simulink model "MdXX_RspToNetWork"  (R2024b)
settings: Solver=FixedStepDiscrete  StartTime=0.0  StopTime=10.0  FixedStep=0.01  RelTol=1e-3
(part 2 of 3)

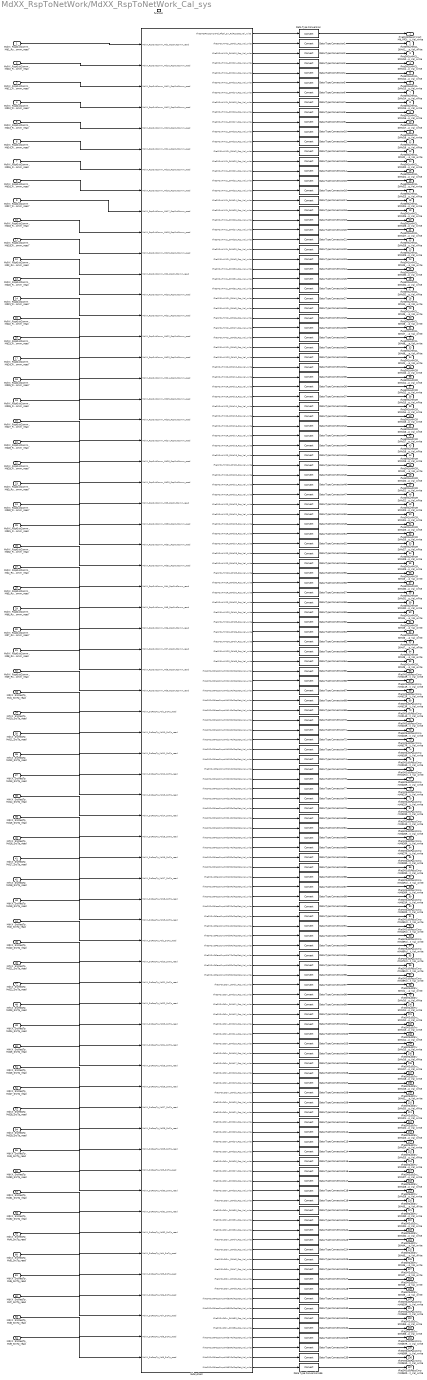
== system MdXX_RspToNetWork/MdXX_RspToNetWork_Cal_sys ==
  MdXX_RspOutComm_Md1_RspOutComm_read : Inport
  MdXX_RspOutComm_Md10_RspOutComm_read : Inport  Port=2
  MdXX_RspOutComm_Md11_RspOutComm_read : Inport  Port=3
  MdXX_RspOutComm_Md12_RspOutComm_read : Inport  Port=4
  MdXX_RspOutComm_Md13_RspOutComm_read : Inport  Port=5
  MdXX_RspOutComm_Md14_RspOutComm_read : Inport  Port=6
  MdXX_RspOutComm_Md15_RspOutComm_read : Inport  Port=7
  MdXX_RspOutComm_Md16_RspOutComm_read : Inport  Port=8
  MdXX_RspOutComm_Md17_RspOutComm_read : Inport  Port=9
  MdXX_RspOutComm_Md18_RspOutComm_read : Inport  Port=10
  MdXX_RspOutComm_Md19_RspOutComm_read : Inport  Port=11
  MdXX_RspOutComm_Md2_RspOutComm_read : Inport  Port=12
  MdXX_RspOutComm_Md20_RspOutComm_read : Inport  Port=13
  MdXX_RspOutComm_Md21_RspOutComm_read : Inport  Port=14
  MdXX_RspOutComm_Md22_RspOutComm_read : Inport  Port=15
  MdXX_RspOutComm_Md23_RspOutComm_read : Inport  Port=16
  MdXX_RspOutComm_Md24_RspOutComm_read : Inport  Port=17
  MdXX_RspOutComm_Md25_RspOutComm_read : Inport  Port=18
  MdXX_RspOutComm_Md26_RspOutComm_read : Inport  Port=19
  MdXX_RspOutComm_Md27_RspOutComm_read : Inport  Port=20
  MdXX_RspOutComm_Md28_RspOutComm_read : Inport  Port=21
  MdXX_RspOutComm_Md29_RspOutComm_read : Inport  Port=22
  MdXX_RspOutComm_Md3_RspOutComm_read : Inport  Port=23
  MdXX_RspOutComm_Md30_RspOutComm_read : Inport  Port=24
  MdXX_RspOutComm_Md31_RspOutComm_read : Inport  Port=25
  MdXX_RspOutComm_Md32_RspOutComm_read : Inport  Port=26
  MdXX_RspOutComm_Md4_RspOutComm_read : Inport  Port=27
  MdXX_RspOutComm_Md5_RspOutComm_read : Inport  Port=28
  MdXX_RspOutComm_Md6_RspOutComm_read : Inport  Port=29
  MdXX_RspOutComm_Md7_RspOutComm_read : Inport  Port=30
  MdXX_RspOutComm_Md8_RspOutComm_read : Inport  Port=31
  MdXX_RspOutComm_Md9_RspOutComm_read : Inport  Port=32
  MdXX_SrcReqTp_Md1_SrcTp_read : Inport  Port=33
  MdXX_SrcReqTp_Md10_SrcTp_read : Inport  Port=34
  MdXX_SrcReqTp_Md11_SrcTp_read : Inport  Port=35
  MdXX_SrcReqTp_Md12_SrcTp_read : Inport  Port=36
  MdXX_SrcReqTp_Md13_SrcTp_read : Inport  Port=37
  MdXX_SrcReqTp_Md14_SrcTp_read : Inport  Port=38
  MdXX_SrcReqTp_Md15_SrcTp_read : Inport  Port=39
  MdXX_SrcReqTp_Md16_SrcTp_read : Inport  Port=40
  MdXX_SrcReqTp_Md17_SrcTp_read : Inport  Port=41
  MdXX_SrcReqTp_Md18_SrcTp_read : Inport  Port=42
  MdXX_SrcReqTp_Md19_SrcTp_read : Inport  Port=43
  MdXX_SrcReqTp_Md2_SrcTp_read : Inport  Port=44
  MdXX_SrcReqTp_Md20_SrcTp_read : Inport  Port=45
  MdXX_SrcReqTp_Md21_SrcTp_read : Inport  Port=46
  MdXX_SrcReqTp_Md22_SrcTp_read : Inport  Port=47
  MdXX_SrcReqTp_Md23_SrcTp_read : Inport  Port=48
  MdXX_SrcReqTp_Md24_SrcTp_read : Inport  Port=49
  MdXX_SrcReqTp_Md25_SrcTp_read : Inport  Port=50
  MdXX_SrcReqTp_Md26_SrcTp_read : Inport  Port=51
  MdXX_SrcReqTp_Md27_SrcTp_read : Inport  Port=52
  MdXX_SrcReqTp_Md28_SrcTp_read : Inport  Port=53
  MdXX_SrcReqTp_Md29_SrcTp_read : Inport  Port=54
  MdXX_SrcReqTp_Md3_SrcTp_read : Inport  Port=55
  MdXX_SrcReqTp_Md30_SrcTp_read : Inport  Port=56
  MdXX_SrcReqTp_Md31_SrcTp_read : Inport  Port=57
  MdXX_SrcReqTp_Md32_SrcTp_read : Inport  Port=58
  MdXX_SrcReqTp_Md4_SrcTp_read : Inport  Port=59
  MdXX_SrcReqTp_Md5_SrcTp_read : Inport  Port=60
  MdXX_SrcReqTp_Md6_SrcTp_read : Inport  Port=61
  MdXX_SrcReqTp_Md7_SrcTp_read : Inport  Port=62
  MdXX_SrcReqTp_Md8_SrcTp_read : Inport  Port=63
  MdXX_SrcReqTp_Md9_SrcTp_read : Inport  Port=64
  function : TriggerPort  TriggerType=function-call  IsSimulinkFunction=on  FunctionName=MdXX_RspToNetWork_Cal  VariantControl=(inherit)
  Data Type Conversion{,1..136} (137 alike) : DataTypeConversion  SaturateOnIntegerOverflow=off  RndMeth=Floor
  Subsystem : Subsystem
  IfVeSMStPassCmprtMd_RfCtrl_Sw_RclRspStat_Val_write : Outport  VectorParamsAs1DForOutWhenUnconnected=off
  IfVeSMSuHMI2L_StMd1_Rsp_Val_write : Outport  Port=2  VectorParamsAs1DForOutWhenUnconnected=off
  IfVeSMSuHMI2L_StMd10_Rsp_Val_write : Outport  Port=3  VectorParamsAs1DForOutWhenUnconnected=off
  IfVeSMSuHMI2L_StMd11_Rsp_Val_write : Outport  Port=4  VectorParamsAs1DForOutWhenUnconnected=off
  IfVeSMSuHMI2L_StMd12_Rsp_Val_write : Outport  Port=5  VectorParamsAs1DForOutWhenUnconnected=off
  IfVeSMSuHMI2L_StMd13_Rsp_Val_write : Outport  Port=6  VectorParamsAs1DForOutWhenUnconnected=off
  IfVeSMSuHMI2L_StMd14_Rsp_Val_write : Outport  Port=7  VectorParamsAs1DForOutWhenUnconnected=off
  IfVeSMSuHMI2L_StMd15_Rsp_Val_write : Outport  Port=8  VectorParamsAs1DForOutWhenUnconnected=off
  IfVeSMSuHMI2L_StMd16_Rsp_Val_write : Outport  Port=9  VectorParamsAs1DForOutWhenUnconnected=off
  IfVeSMSuHMI2L_StMd17_Rsp_Val_write : Outport  Port=10  VectorParamsAs1DForOutWhenUnconnected=off
  IfVeSMSuHMI2L_StMd18_Rsp_Val_write : Outport  Port=11  VectorParamsAs1DForOutWhenUnconnected=off
  IfVeSMSuHMI2L_StMd19_Rsp_Val_write : Outport  Port=12  VectorParamsAs1DForOutWhenUnconnected=off
  IfVeSMSuHMI2L_StMd2_Rsp_Val_write : Outport  Port=13  VectorParamsAs1DForOutWhenUnconnected=off
  IfVeSMSuHMI2L_StMd20_Rsp_Val_write : Outport  Port=14  VectorParamsAs1DForOutWhenUnconnected=off
  IfVeSMSuHMI2L_StMd21_Rsp_Val_write : Outport  Port=15  VectorParamsAs1DForOutWhenUnconnected=off
  IfVeSMSuHMI2L_StMd22_Rsp_Val_write : Outport  Port=16  VectorParamsAs1DForOutWhenUnconnected=off
  IfVeSMSuHMI2L_StMd23_Rsp_Val_write : Outport  Port=17  VectorParamsAs1DForOutWhenUnconnected=off
  IfVeSMSuHMI2L_StMd24_Rsp_Val_write : Outport  Port=18  VectorParamsAs1DForOutWhenUnconnected=off
  IfVeSMSuHMI2L_StMd25_Rsp_Val_write : Outport  Port=19  VectorParamsAs1DForOutWhenUnconnected=off
  IfVeSMSuHMI2L_StMd26_Rsp_Val_write : Outport  Port=20  VectorParamsAs1DForOutWhenUnconnected=off
  IfVeSMSuHMI2L_StMd27_Rsp_Val_write : Outport  Port=21  VectorParamsAs1DForOutWhenUnconnected=off
  IfVeSMSuHMI2L_StMd28_Rsp_Val_write : Outport  Port=22  VectorParamsAs1DForOutWhenUnconnected=off
  IfVeSMSuHMI2L_StMd29_Rsp_Val_write : Outport  Port=23  VectorParamsAs1DForOutWhenUnconnected=off
  IfVeSMSuHMI2L_StMd3_Rsp_Val_write : Outport  Port=24  VectorParamsAs1DForOutWhenUnconnected=off
  IfVeSMSuHMI2L_StMd30_Rsp_Val_write : Outport  Port=25  VectorParamsAs1DForOutWhenUnconnected=off
  IfVeSMSuHMI2L_StMd31_Rsp_Val_write : Outport  Port=26  VectorParamsAs1DForOutWhenUnconnected=off
  IfVeSMSuHMI2L_StMd32_Rsp_Val_write : Outport  Port=27  VectorParamsAs1DForOutWhenUnconnected=off
  IfVeSMSuHMI2L_StMd4_Rsp_Val_write : Outport  Port=28  VectorParamsAs1DForOutWhenUnconnected=off
  IfVeSMSuHMI2L_StMd5_Rsp_Val_write : Outport  Port=29  VectorParamsAs1DForOutWhenUnconnected=off
  IfVeSMSuHMI2L_StMd6_Rsp_Val_write : Outport  Port=30  VectorParamsAs1DForOutWhenUnconnected=off
  IfVeSMSuHMI2L_StMd7_Rsp_Val_write : Outport  Port=31  VectorParamsAs1DForOutWhenUnconnected=off
  IfVeSMSuHMI2L_StMd8_Rsp_Val_write : Outport  Port=32  VectorParamsAs1DForOutWhenUnconnected=off
  IfVeSMSuHMI2L_StMd9_Rsp_Val_write : Outport  Port=33  VectorParamsAs1DForOutWhenUnconnected=off
  IfVeSMSuHMI2R_StMd1_Rsp_Val_write : Outport  Port=34  VectorParamsAs1DForOutWhenUnconnected=off
  IfVeSMSuHMI2R_StMd10_Rsp_Val_write : Outport  Port=35  VectorParamsAs1DForOutWhenUnconnected=off
  IfVeSMSuHMI2R_StMd11_Rsp_Val_write : Outport  Port=36  VectorParamsAs1DForOutWhenUnconnected=off
  IfVeSMSuHMI2R_StMd12_Rsp_Val_write : Outport  Port=37  VectorParamsAs1DForOutWhenUnconnected=off
  IfVeSMSuHMI2R_StMd13_Rsp_Val_write : Outport  Port=38  VectorParamsAs1DForOutWhenUnconnected=off
  IfVeSMSuHMI2R_StMd14_Rsp_Val_write : Outport  Port=39  VectorParamsAs1DForOutWhenUnconnected=off
  IfVeSMSuHMI2R_StMd15_Rsp_Val_write : Outport  Port=40  VectorParamsAs1DForOutWhenUnconnected=off
  IfVeSMSuHMI2R_StMd16_Rsp_Val_write : Outport  Port=41  VectorParamsAs1DForOutWhenUnconnected=off
  IfVeSMSuHMI2R_StMd17_Rsp_Val_write : Outport  Port=42  VectorParamsAs1DForOutWhenUnconnected=off
  IfVeSMSuHMI2R_StMd18_Rsp_Val_write : Outport  Port=43  VectorParamsAs1DForOutWhenUnconnected=off
  IfVeSMSuHMI2R_StMd19_Rsp_Val_write : Outport  Port=44  VectorParamsAs1DForOutWhenUnconnected=off
  IfVeSMSuHMI2R_StMd2_Rsp_Val_write : Outport  Port=45  VectorParamsAs1DForOutWhenUnconnected=off
  IfVeSMSuHMI2R_StMd20_Rsp_Val_write : Outport  Port=46  VectorParamsAs1DForOutWhenUnconnected=off
  IfVeSMSuHMI2R_StMd21_Rsp_Val_write : Outport  Port=47  VectorParamsAs1DForOutWhenUnconnected=off
  IfVeSMSuHMI2R_StMd22_Rsp_Val_write : Outport  Port=48  VectorParamsAs1DForOutWhenUnconnected=off
  IfVeSMSuHMI2R_StMd23_Rsp_Val_write : Outport  Port=49  VectorParamsAs1DForOutWhenUnconnected=off
  IfVeSMSuHMI2R_StMd24_Rsp_Val_write : Outport  Port=50  VectorParamsAs1DForOutWhenUnconnected=off
  IfVeSMSuHMI2R_StMd25_Rsp_Val_write : Outport  Port=51  VectorParamsAs1DForOutWhenUnconnected=off
  IfVeSMSuHMI2R_StMd26_Rsp_Val_write : Outport  Port=52  VectorParamsAs1DForOutWhenUnconnected=off
  IfVeSMSuHMI2R_StMd27_Rsp_Val_write : Outport  Port=53  VectorParamsAs1DForOutWhenUnconnected=off
  IfVeSMSuHMI2R_StMd28_Rsp_Val_write : Outport  Port=54  VectorParamsAs1DForOutWhenUnconnected=off
  IfVeSMSuHMI2R_StMd29_Rsp_Val_write : Outport  Port=55  VectorParamsAs1DForOutWhenUnconnected=off
  IfVeSMSuHMI2R_StMd3_Rsp_Val_write : Outport  Port=56  VectorParamsAs1DForOutWhenUnconnected=off
  IfVeSMSuHMI2R_StMd30_Rsp_Val_write : Outport  Port=57  VectorParamsAs1DForOutWhenUnconnected=off
  IfVeSMSuHMI2R_StMd31_Rsp_Val_write : Outport  Port=58  VectorParamsAs1DForOutWhenUnconnected=off
  IfVeSMSuHMI2R_StMd32_Rsp_Val_write : Outport  Port=59  VectorParamsAs1DForOutWhenUnconnected=off
  IfVeSMSuHMI2R_StMd4_Rsp_Val_write : Outport  Port=60  VectorParamsAs1DForOutWhenUnconnected=off
  IfVeSMSuHMI2R_StMd5_Rsp_Val_write : Outport  Port=61  VectorParamsAs1DForOutWhenUnconnected=off
  IfVeSMSuHMI2R_StMd6_Rsp_Val_write : Outport  Port=62  VectorParamsAs1DForOutWhenUnconnected=off
  IfVeSMSuHMI2R_StMd7_Rsp_Val_write : Outport  Port=63  VectorParamsAs1DForOutWhenUnconnected=off
  IfVeSMSuHMI2R_StMd8_Rsp_Val_write : Outport  Port=64  VectorParamsAs1DForOutWhenUnconnected=off
  IfVeSMSuHMI2R_StMd9_Rsp_Val_write : Outport  Port=65  VectorParamsAs1DForOutWhenUnconnected=off
  IfVeSMSuStPassCmprtMd10RclRspStat_Val_write : Outport  Port=66  VectorParamsAs1DForOutWhenUnconnected=off
  IfVeSMSuStPassCmprtMd11RclRspStat_Val_write : Outport  Port=67  VectorParamsAs1DForOutWhenUnconnected=off
  IfVeSMSuStPassCmprtMd12RclRspStat_Val_write : Outport  Port=68  VectorParamsAs1DForOutWhenUnconnected=off
  IfVeSMSuStPassCmprtMd13RclRspStat_Val_write : Outport  Port=69  VectorParamsAs1DForOutWhenUnconnected=off
  IfVeSMSuStPassCmprtMd14RclRspStat_Val_write : Outport  Port=70  VectorParamsAs1DForOutWhenUnconnected=off
  IfVeSMSuStPassCmprtMd15RclRspStat_Val_write : Outport  Port=71  VectorParamsAs1DForOutWhenUnconnected=off
  IfVeSMSuStPassCmprtMd16RclRspStat_Val_write : Outport  Port=72  VectorParamsAs1DForOutWhenUnconnected=off
  IfVeSMSuStPassCmprtMd17RclRspStat_Val_write : Outport  Port=73  VectorParamsAs1DForOutWhenUnconnected=off
  IfVeSMSuStPassCmprtMd18RclRspStat_Val_write : Outport  Port=74  VectorParamsAs1DForOutWhenUnconnected=off
  IfVeSMSuStPassCmprtMd19RclRspStat_Val_write : Outport  Port=75  VectorParamsAs1DForOutWhenUnconnected=off
  IfVeSMSuStPassCmprtMd1RclRspStat_Val_write : Outport  Port=76  VectorParamsAs1DForOutWhenUnconnected=off
  IfVeSMSuStPassCmprtMd20RclRspStat_Val_write : Outport  Port=77  VectorParamsAs1DForOutWhenUnconnected=off
  IfVeSMSuStPassCmprtMd21RclRspStat_Val_write : Outport  Port=78  VectorParamsAs1DForOutWhenUnconnected=off
  IfVeSMSuStPassCmprtMd22RclRspStat_Val_write : Outport  Port=79  VectorParamsAs1DForOutWhenUnconnected=off
  IfVeSMSuStPassCmprtMd23RclRspStat_Val_write : Outport  Port=80  VectorParamsAs1DForOutWhenUnconnected=off
  IfVeSMSuStPassCmprtMd24RclRspStat_Val_write : Outport  Port=81  VectorParamsAs1DForOutWhenUnconnected=off
  IfVeSMSuStPassCmprtMd25RclRspStat_Val_write : Outport  Port=82  VectorParamsAs1DForOutWhenUnconnected=off
  IfVeSMSuStPassCmprtMd26RclRspStat_Val_write : Outport  Port=83  VectorParamsAs1DForOutWhenUnconnected=off
  IfVeSMSuStPassCmprtMd27RclRspStat_Val_write : Outport  Port=84  VectorParamsAs1DForOutWhenUnconnected=off
  IfVeSMSuStPassCmprtMd28RclRspStat_Val_write : Outport  Port=85  VectorParamsAs1DForOutWhenUnconnected=off
  IfVeSMSuStPassCmprtMd29RclRspStat_Val_write : Outport  Port=86  VectorParamsAs1DForOutWhenUnconnected=off
  IfVeSMSuStPassCmprtMd2RclRspStat_Val_write : Outport  Port=87  VectorParamsAs1DForOutWhenUnconnected=off
  IfVeSMSuStPassCmprtMd30RclRspStat_Val_write : Outport  Port=88  VectorParamsAs1DForOutWhenUnconnected=off
  IfVeSMSuStPassCmprtMd31RclRspStat_Val_write : Outport  Port=89  VectorParamsAs1DForOutWhenUnconnected=off
  IfVeSMSuStPassCmprtMd32RclRspStat_Val_write : Outport  Port=90  VectorParamsAs1DForOutWhenUnconnected=off
  IfVeSMSuStPassCmprtMd3RclRspStat_Val_write : Outport  Port=91  VectorParamsAs1DForOutWhenUnconnected=off
  IfVeSMSuStPassCmprtMd4RclRspStat_Val_write : Outport  Port=92  VectorParamsAs1DForOutWhenUnconnected=off
  IfVeSMSuStPassCmprtMd5RclRspStat_Val_write : Outport  Port=93  VectorParamsAs1DForOutWhenUnconnected=off
  IfVeSMSuStPassCmprtMd6RclRspStat_Val_write : Outport  Port=94  VectorParamsAs1DForOutWhenUnconnected=off
  IfVeSMSuStPassCmprtMd7RclRspStat_Val_write : Outport  Port=95  VectorParamsAs1DForOutWhenUnconnected=off
  IfVeSMSuStPassCmprtMd8RclRspStat_Val_write : Outport  Port=96  VectorParamsAs1DForOutWhenUnconnected=off
  IfVeSMSuStPassCmprtMd9RclRspStat_Val_write : Outport  Port=97  VectorParamsAs1DForOutWhenUnconnected=off
  IfVeSMSuStSrv_StMd1_Rsp_Val_write : Outport  Port=98  VectorParamsAs1DForOutWhenUnconnected=off
  IfVeSMSuStSrv_StMd10_Rsp_Val_write : Outport  Port=99  VectorParamsAs1DForOutWhenUnconnected=off
  IfVeSMSuStSrv_StMd11_Rsp_Val_write : Outport  Port=100  VectorParamsAs1DForOutWhenUnconnected=off
  IfVeSMSuStSrv_StMd12_Rsp_Val_write : Outport  Port=101  VectorParamsAs1DForOutWhenUnconnected=off
  IfVeSMSuStSrv_StMd13_Rsp_Val_write : Outport  Port=102  VectorParamsAs1DForOutWhenUnconnected=off
  IfVeSMSuStSrv_StMd14_Rsp_Val_write : Outport  Port=103  VectorParamsAs1DForOutWhenUnconnected=off
  IfVeSMSuStSrv_StMd15_Rsp_Val_write : Outport  Port=104  VectorParamsAs1DForOutWhenUnconnected=off
  IfVeSMSuStSrv_StMd16_Rsp_Val_write : Outport  Port=105  VectorParamsAs1DForOutWhenUnconnected=off
  IfVeSMSuStSrv_StMd17_Rsp_Val_write : Outport  Port=106  VectorParamsAs1DForOutWhenUnconnected=off
  IfVeSMSuStSrv_StMd18_Rsp_Val_write : Outport  Port=107  VectorParamsAs1DForOutWhenUnconnected=off
  IfVeSMSuStSrv_StMd19_Rsp_Val_write : Outport  Port=108  VectorParamsAs1DForOutWhenUnconnected=off
  IfVeSMSuStSrv_StMd2_Rsp_Val_write : Outport  Port=109  VectorParamsAs1DForOutWhenUnconnected=off
  IfVeSMSuStSrv_StMd20_Rsp_Val_write : Outport  Port=110  VectorParamsAs1DForOutWhenUnconnected=off
  IfVeSMSuStSrv_StMd21_Rsp_Val_write : Outport  Port=111  VectorParamsAs1DForOutWhenUnconnected=off
  IfVeSMSuStSrv_StMd22_Rsp_Val_write : Outport  Port=112  VectorParamsAs1DForOutWhenUnconnected=off
  IfVeSMSuStSrv_StMd23_Rsp_Val_write : Outport  Port=113  VectorParamsAs1DForOutWhenUnconnected=off
  IfVeSMSuStSrv_StMd24_Rsp_Val_write : Outport  Port=114  VectorParamsAs1DForOutWhenUnconnected=off
  IfVeSMSuStSrv_StMd25_Rsp_Val_write : Outport  Port=115  VectorParamsAs1DForOutWhenUnconnected=off
  IfVeSMSuStSrv_StMd26_Rsp_Val_write : Outport  Port=116  VectorParamsAs1DForOutWhenUnconnected=off
  IfVeSMSuStSrv_StMd27_Rsp_Val_write : Outport  Port=117  VectorParamsAs1DForOutWhenUnconnected=off
  IfVeSMSuStSrv_StMd28_Rsp_Val_write : Outport  Port=118  VectorParamsAs1DForOutWhenUnconnected=off
  IfVeSMSuStSrv_StMd29_Rsp_Val_write : Outport  Port=119  VectorParamsAs1DForOutWhenUnconnected=off
  IfVeSMSuStSrv_StMd3_Rsp_Val_write : Outport  Port=120  VectorParamsAs1DForOutWhenUnconnected=off
  IfVeSMSuStSrv_StMd30_Rsp_Val_write : Outport  Port=121  VectorParamsAs1DForOutWhenUnconnected=off
  IfVeSMSuStSrv_StMd31_Rsp_Val_write : Outport  Port=122  VectorParamsAs1DForOutWhenUnconnected=off
  IfVeSMSuStSrv_StMd32_Rsp_Val_write : Outport  Port=123  VectorParamsAs1DForOutWhenUnconnected=off
  IfVeSMSuStSrv_StMd4_Rsp_Val_write : Outport  Port=124  VectorParamsAs1DForOutWhenUnconnected=off
  IfVeSMSuStSrv_StMd5_Rsp_Val_write : Outport  Port=125  VectorParamsAs1DForOutWhenUnconnected=off
  IfVeSMSuStSrv_StMd6_Rsp_Val_write : Outport  Port=126  VectorParamsAs1DForOutWhenUnconnected=off
  IfVeSMSuStSrv_StMd7_Rsp_Val_write : Outport  Port=127  VectorParamsAs1DForOutWhenUnconnected=off
  IfVeSMSuStSrv_StMd8_Rsp_Val_write : Outport  Port=128  VectorParamsAs1DForOutWhenUnconnected=off
  IfVeSMSuStSrv_StMd9_Rsp_Val_write : Outport  Port=129  VectorParamsAs1DForOutWhenUnconnected=off
  IfVeSMSuStPassCmprtMd53RclRspStat_Val_write : Outport  Port=130  VectorParamsAs1DForOutWhenUnconnected=off
  IfVeSMSuStPassCmprtMd56RclRspStat_Val_write : Outport  Port=131  VectorParamsAs1DForOutWhenUnconnected=off
  IfVeSMSuStSrv_StMd53_Rsp_Val_write : Outport  Port=132  VectorParamsAs1DForOutWhenUnconnected=off
  IfVeSMSuStSrv_StMd56_Rsp_Val_write : Outport  Port=133  VectorParamsAs1DForOutWhenUnconnected=off
  IfVeSMSuStPassCmprtMd57RclRspStat_Val_write : Outport  Port=134  VectorParamsAs1DForOutWhenUnconnected=off
      settings: EnsureOutportIsVirtual=on
  IfVeSMSuStPassCmprtMd58RclRspStat_Val_write : Outport  Port=135  VectorParamsAs1DForOutWhenUnconnected=off
      settings: EnsureOutportIsVirtual=on
  IfVeSMSuStPassCmprtMd61RclRspStat_Val_write : Outport  Port=136  VectorParamsAs1DForOutWhenUnconnected=off
      settings: EnsureOutportIsVirtual=on
  IfVeSMSuStPassCmprtMd62RclRspStat_Val_write : Outport  Port=137  VectorParamsAs1DForOutWhenUnconnected=off
      settings: EnsureOutportIsVirtual=on
  wires:
  MdXX_RspOutComm_Md1_RspOutComm_read/1 -> Subsystem/1(MdXX_RspOutComm_Md1_RspOutComm_read)
  MdXX_RspOutComm_Md10_RspOutComm_read/1 -> Subsystem/2(MdXX_RspOutComm_Md10_RspOutComm_read)
  MdXX_RspOutComm_Md11_RspOutComm_read/1 -> Subsystem/3(MdXX_RspOutComm_Md11_RspOutComm_read)
  MdXX_RspOutComm_Md12_RspOutComm_read/1 -> Subsystem/4(MdXX_RspOutComm_Md12_RspOutComm_read)
  MdXX_RspOutComm_Md13_RspOutComm_read/1 -> Subsystem/5(MdXX_RspOutComm_Md13_RspOutComm_read)
  MdXX_RspOutComm_Md14_RspOutComm_read/1 -> Subsystem/6(MdXX_RspOutComm_Md14_RspOutComm_read)
  MdXX_RspOutComm_Md15_RspOutComm_read/1 -> Subsystem/7(MdXX_RspOutComm_Md15_RspOutComm_read)
  MdXX_RspOutComm_Md16_RspOutComm_read/1 -> Subsystem/8(MdXX_RspOutComm_Md16_RspOutComm_read)
  MdXX_RspOutComm_Md17_RspOutComm_read/1 -> Subsystem/9(MdXX_RspOutComm_Md17_RspOutComm_read)
  MdXX_RspOutComm_Md18_RspOutComm_read/1 -> Subsystem/10(MdXX_RspOutComm_Md18_RspOutComm_read)
  MdXX_RspOutComm_Md19_RspOutComm_read/1 -> Subsystem/11(MdXX_RspOutComm_Md19_RspOutComm_read)
  MdXX_RspOutComm_Md2_RspOutComm_read/1 -> Subsystem/12(MdXX_RspOutComm_Md2_RspOutComm_read)
  MdXX_RspOutComm_Md20_RspOutComm_read/1 -> Subsystem/13(MdXX_RspOutComm_Md20_RspOutComm_read)
  MdXX_RspOutComm_Md21_RspOutComm_read/1 -> Subsystem/14(MdXX_RspOutComm_Md21_RspOutComm_read)
  MdXX_RspOutComm_Md22_RspOutComm_read/1 -> Subsystem/15(MdXX_RspOutComm_Md22_RspOutComm_read)
  MdXX_RspOutComm_Md23_RspOutComm_read/1 -> Subsystem/16(MdXX_RspOutComm_Md23_RspOutComm_read)
  MdXX_RspOutComm_Md24_RspOutComm_read/1 -> Subsystem/17(MdXX_RspOutComm_Md24_RspOutComm_read)
  MdXX_RspOutComm_Md25_RspOutComm_read/1 -> Subsystem/18(MdXX_RspOutComm_Md25_RspOutComm_read)
  MdXX_RspOutComm_Md26_RspOutComm_read/1 -> Subsystem/19(MdXX_RspOutComm_Md26_RspOutComm_read)
  MdXX_RspOutComm_Md27_RspOutComm_read/1 -> Subsystem/20(MdXX_RspOutComm_Md27_RspOutComm_read)
  MdXX_RspOutComm_Md28_RspOutComm_read/1 -> Subsystem/21(MdXX_RspOutComm_Md28_RspOutComm_read)
  MdXX_RspOutComm_Md29_RspOutComm_read/1 -> Subsystem/22(MdXX_RspOutComm_Md29_RspOutComm_read)
  MdXX_RspOutComm_Md3_RspOutComm_read/1 -> Subsystem/23(MdXX_RspOutComm_Md3_RspOutComm_read)
  MdXX_RspOutComm_Md30_RspOutComm_read/1 -> Subsystem/24(MdXX_RspOutComm_Md30_RspOutComm_read)
  MdXX_RspOutComm_Md31_RspOutComm_read/1 -> Subsystem/25(MdXX_RspOutComm_Md31_RspOutComm_read)
  MdXX_RspOutComm_Md32_RspOutComm_read/1 -> Subsystem/26(MdXX_RspOutComm_Md32_RspOutComm_read)
  MdXX_RspOutComm_Md4_RspOutComm_read/1 -> Subsystem/27(MdXX_RspOutComm_Md4_RspOutComm_read)
  MdXX_RspOutComm_Md5_RspOutComm_read/1 -> Subsystem/28(MdXX_RspOutComm_Md5_RspOutComm_read)
  MdXX_RspOutComm_Md6_RspOutComm_read/1 -> Subsystem/29(MdXX_RspOutComm_Md6_RspOutComm_read)
  MdXX_RspOutComm_Md7_RspOutComm_read/1 -> Subsystem/30(MdXX_RspOutComm_Md7_RspOutComm_read)
  MdXX_RspOutComm_Md8_RspOutComm_read/1 -> Subsystem/31(MdXX_RspOutComm_Md8_RspOutComm_read)
  MdXX_RspOutComm_Md9_RspOutComm_read/1 -> Subsystem/32(MdXX_RspOutComm_Md9_RspOutComm_read)
  MdXX_SrcReqTp_Md1_SrcTp_read/1 -> Subsystem/33(MdXX_SrcReqTp_Md1_SrcTp_read)
  MdXX_SrcReqTp_Md10_SrcTp_read/1 -> Subsystem/34(MdXX_SrcReqTp_Md10_SrcTp_read)
  MdXX_SrcReqTp_Md11_SrcTp_read/1 -> Subsystem/35(MdXX_SrcReqTp_Md11_SrcTp_read)
  MdXX_SrcReqTp_Md12_SrcTp_read/1 -> Subsystem/36(MdXX_SrcReqTp_Md12_SrcTp_read)
  MdXX_SrcReqTp_Md13_SrcTp_read/1 -> Subsystem/37(MdXX_SrcReqTp_Md13_SrcTp_read)
  MdXX_SrcReqTp_Md14_SrcTp_read/1 -> Subsystem/38(MdXX_SrcReqTp_Md14_SrcTp_read)
  MdXX_SrcReqTp_Md15_SrcTp_read/1 -> Subsystem/39(MdXX_SrcReqTp_Md15_SrcTp_read)
  MdXX_SrcReqTp_Md16_SrcTp_read/1 -> Subsystem/40(MdXX_SrcReqTp_Md16_SrcTp_read)
  MdXX_SrcReqTp_Md17_SrcTp_read/1 -> Subsystem/41(MdXX_SrcReqTp_Md17_SrcTp_read)
  MdXX_SrcReqTp_Md18_SrcTp_read/1 -> Subsystem/42(MdXX_SrcReqTp_Md18_SrcTp_read)
  MdXX_SrcReqTp_Md19_SrcTp_read/1 -> Subsystem/43(MdXX_SrcReqTp_Md19_SrcTp_read)
  MdXX_SrcReqTp_Md2_SrcTp_read/1 -> Subsystem/44(MdXX_SrcReqTp_Md2_SrcTp_read)
  MdXX_SrcReqTp_Md20_SrcTp_read/1 -> Subsystem/45(MdXX_SrcReqTp_Md20_SrcTp_read)
  MdXX_SrcReqTp_Md21_SrcTp_read/1 -> Subsystem/46(MdXX_SrcReqTp_Md21_SrcTp_read)
  MdXX_SrcReqTp_Md22_SrcTp_read/1 -> Subsystem/47(MdXX_SrcReqTp_Md22_SrcTp_read)
  MdXX_SrcReqTp_Md23_SrcTp_read/1 -> Subsystem/48(MdXX_SrcReqTp_Md23_SrcTp_read)
  MdXX_SrcReqTp_Md24_SrcTp_read/1 -> Subsystem/49(MdXX_SrcReqTp_Md24_SrcTp_read)
  MdXX_SrcReqTp_Md25_SrcTp_read/1 -> Subsystem/50(MdXX_SrcReqTp_Md25_SrcTp_read)
  MdXX_SrcReqTp_Md26_SrcTp_read/1 -> Subsystem/51(MdXX_SrcReqTp_Md26_SrcTp_read)
  MdXX_SrcReqTp_Md27_SrcTp_read/1 -> Subsystem/52(MdXX_SrcReqTp_Md27_SrcTp_read)
  MdXX_SrcReqTp_Md28_SrcTp_read/1 -> Subsystem/53(MdXX_SrcReqTp_Md28_SrcTp_read)
  MdXX_SrcReqTp_Md29_SrcTp_read/1 -> Subsystem/54(MdXX_SrcReqTp_Md29_SrcTp_read)
  MdXX_SrcReqTp_Md3_SrcTp_read/1 -> Subsystem/55(MdXX_SrcReqTp_Md3_SrcTp_read)
  MdXX_SrcReqTp_Md30_SrcTp_read/1 -> Subsystem/56(MdXX_SrcReqTp_Md30_SrcTp_read)
  MdXX_SrcReqTp_Md31_SrcTp_read/1 -> Subsystem/57(MdXX_SrcReqTp_Md31_SrcTp_read)
  MdXX_SrcReqTp_Md32_SrcTp_read/1 -> Subsystem/58(MdXX_SrcReqTp_Md32_SrcTp_read)
  MdXX_SrcReqTp_Md4_SrcTp_read/1 -> Subsystem/59(MdXX_SrcReqTp_Md4_SrcTp_read)
  MdXX_SrcReqTp_Md5_SrcTp_read/1 -> Subsystem/60(MdXX_SrcReqTp_Md5_SrcTp_read)
  MdXX_SrcReqTp_Md6_SrcTp_read/1 -> Subsystem/61(MdXX_SrcReqTp_Md6_SrcTp_read)
  MdXX_SrcReqTp_Md7_SrcTp_read/1 -> Subsystem/62(MdXX_SrcReqTp_Md7_SrcTp_read)
  MdXX_SrcReqTp_Md8_SrcTp_read/1 -> Subsystem/63(MdXX_SrcReqTp_Md8_SrcTp_read)
  MdXX_SrcReqTp_Md9_SrcTp_read/1 -> Subsystem/64(MdXX_SrcReqTp_Md9_SrcTp_read)
  Subsystem/1(IfVeSMStPassCmprtMd_RfCtrl_Sw_RclRspStat_Val_write) -> Data Type Conversion/1
  Subsystem/2(IfVeSMSuHMI2L_StMd1_Rsp_Val_write) -> Data Type Conversion1/1
  Subsystem/3(IfVeSMSuHMI2L_StMd10_Rsp_Val_write) -> Data Type Conversion2/1
  Subsystem/4(IfVeSMSuHMI2L_StMd11_Rsp_Val_write) -> Data Type Conversion3/1
  Subsystem/5(IfVeSMSuHMI2L_StMd12_Rsp_Val_write) -> Data Type Conversion4/1
  Subsystem/6(IfVeSMSuHMI2L_StMd13_Rsp_Val_write) -> Data Type Conversion5/1
  Subsystem/7(IfVeSMSuHMI2L_StMd14_Rsp_Val_write) -> Data Type Conversion6/1
  Subsystem/8(IfVeSMSuHMI2L_StMd15_Rsp_Val_write) -> Data Type Conversion7/1
  Subsystem/9(IfVeSMSuHMI2L_StMd16_Rsp_Val_write) -> Data Type Conversion8/1
  Subsystem/10(IfVeSMSuHMI2L_StMd17_Rsp_Val_write) -> Data Type Conversion9/1
  Subsystem/11(IfVeSMSuHMI2L_StMd18_Rsp_Val_write) -> Data Type Conversion10/1
  Subsystem/12(IfVeSMSuHMI2L_StMd19_Rsp_Val_write) -> Data Type Conversion12/1
  Subsystem/13(IfVeSMSuHMI2L_StMd2_Rsp_Val_write) -> Data Type Conversion11/1
  Subsystem/14(IfVeSMSuHMI2L_StMd20_Rsp_Val_write) -> Data Type Conversion13/1
  Subsystem/15(IfVeSMSuHMI2L_StMd21_Rsp_Val_write) -> Data Type Conversion14/1
  Subsystem/16(IfVeSMSuHMI2L_StMd22_Rsp_Val_write) -> Data Type Conversion15/1
  Subsystem/17(IfVeSMSuHMI2L_StMd23_Rsp_Val_write) -> Data Type Conversion16/1
  Subsystem/18(IfVeSMSuHMI2L_StMd24_Rsp_Val_write) -> Data Type Conversion17/1
  Subsystem/19(IfVeSMSuHMI2L_StMd25_Rsp_Val_write) -> Data Type Conversion18/1
  Subsystem/20(IfVeSMSuHMI2L_StMd26_Rsp_Val_write) -> Data Type Conversion19/1
  Subsystem/21(IfVeSMSuHMI2L_StMd27_Rsp_Val_write) -> Data Type Conversion20/1
  Subsystem/22(IfVeSMSuHMI2L_StMd28_Rsp_Val_write) -> Data Type Conversion21/1
  Subsystem/23(IfVeSMSuHMI2L_StMd29_Rsp_Val_write) -> Data Type Conversion22/1
  Subsystem/24(IfVeSMSuHMI2L_StMd3_Rsp_Val_write) -> Data Type Conversion23/1
  Subsystem/25(IfVeSMSuHMI2L_StMd30_Rsp_Val_write) -> Data Type Conversion24/1
  Subsystem/26(IfVeSMSuHMI2L_StMd31_Rsp_Val_write) -> Data Type Conversion25/1
  Subsystem/27(IfVeSMSuHMI2L_StMd32_Rsp_Val_write) -> Data Type Conversion26/1
  Subsystem/28(IfVeSMSuHMI2L_StMd4_Rsp_Val_write) -> Data Type Conversion27/1
  Subsystem/29(IfVeSMSuHMI2L_StMd5_Rsp_Val_write) -> Data Type Conversion28/1
  Subsystem/30(IfVeSMSuHMI2L_StMd6_Rsp_Val_write) -> Data Type Conversion29/1
  Subsystem/31(IfVeSMSuHMI2L_StMd7_Rsp_Val_write) -> Data Type Conversion30/1
  Subsystem/32(IfVeSMSuHMI2L_StMd8_Rsp_Val_write) -> Data Type Conversion31/1
  Subsystem/33(IfVeSMSuHMI2L_StMd9_Rsp_Val_write) -> Data Type Conversion32/1
  Subsystem/34(IfVeSMSuHMI2R_StMd1_Rsp_Val_write) -> Data Type Conversion33/1
  Subsystem/35(IfVeSMSuHMI2R_StMd10_Rsp_Val_write) -> Data Type Conversion34/1
  Subsystem/36(IfVeSMSuHMI2R_StMd11_Rsp_Val_write) -> Data Type Conversion35/1
  Subsystem/37(IfVeSMSuHMI2R_StMd12_Rsp_Val_write) -> Data Type Conversion36/1
  Subsystem/38(IfVeSMSuHMI2R_StMd13_Rsp_Val_write) -> Data Type Conversion37/1
  Subsystem/39(IfVeSMSuHMI2R_StMd14_Rsp_Val_write) -> Data Type Conversion38/1
  Subsystem/40(IfVeSMSuHMI2R_StMd15_Rsp_Val_write) -> Data Type Conversion39/1
  Subsystem/41(IfVeSMSuHMI2R_StMd16_Rsp_Val_write) -> Data Type Conversion40/1
  Subsystem/42(IfVeSMSuHMI2R_StMd17_Rsp_Val_write) -> Data Type Conversion41/1
  Subsystem/43(IfVeSMSuHMI2R_StMd18_Rsp_Val_write) -> Data Type Conversion42/1
  Subsystem/44(IfVeSMSuHMI2R_StMd19_Rsp_Val_write) -> Data Type Conversion43/1
  Subsystem/45(IfVeSMSuHMI2R_StMd2_Rsp_Val_write) -> Data Type Conversion44/1
  Subsystem/46(IfVeSMSuHMI2R_StMd20_Rsp_Val_write) -> Data Type Conversion45/1
  Subsystem/47(IfVeSMSuHMI2R_StMd21_Rsp_Val_write) -> Data Type Conversion46/1
  Subsystem/48(IfVeSMSuHMI2R_StMd22_Rsp_Val_write) -> Data Type Conversion47/1
  Subsystem/49(IfVeSMSuHMI2R_StMd23_Rsp_Val_write) -> Data Type Conversion48/1
  Subsystem/50(IfVeSMSuHMI2R_StMd24_Rsp_Val_write) -> Data Type Conversion50/1
  Subsystem/51(IfVeSMSuHMI2R_StMd25_Rsp_Val_write) -> Data Type Conversion49/1
  Subsystem/52(IfVeSMSuHMI2R_StMd26_Rsp_Val_write) -> Data Type Conversion51/1
  Subsystem/53(IfVeSMSuHMI2R_StMd27_Rsp_Val_write) -> Data Type Conversion52/1
  Subsystem/54(IfVeSMSuHMI2R_StMd28_Rsp_Val_write) -> Data Type Conversion53/1
  Subsystem/55(IfVeSMSuHMI2R_StMd29_Rsp_Val_write) -> Data Type Conversion54/1
  Subsystem/56(IfVeSMSuHMI2R_StMd3_Rsp_Val_write) -> Data Type Conversion55/1
  Subsystem/57(IfVeSMSuHMI2R_StMd30_Rsp_Val_write) -> Data Type Conversion56/1
  Subsystem/58(IfVeSMSuHMI2R_StMd31_Rsp_Val_write) -> Data Type Conversion57/1
  Subsystem/59(IfVeSMSuHMI2R_StMd32_Rsp_Val_write) -> Data Type Conversion58/1
  Subsystem/60(IfVeSMSuHMI2R_StMd4_Rsp_Val_write) -> Data Type Conversion59/1
  Subsystem/61(IfVeSMSuHMI2R_StMd5_Rsp_Val_write) -> Data Type Conversion60/1
  Subsystem/62(IfVeSMSuHMI2R_StMd6_Rsp_Val_write) -> Data Type Conversion61/1
  Subsystem/63(IfVeSMSuHMI2R_StMd7_Rsp_Val_write) -> Data Type Conversion62/1
  Subsystem/64(IfVeSMSuHMI2R_StMd8_Rsp_Val_write) -> Data Type Conversion63/1
  Subsystem/65(IfVeSMSuHMI2R_StMd9_Rsp_Val_write) -> Data Type Conversion64/1
  Subsystem/66(IfVeSMSuStPassCmprtMd10RclRspStat_Val_write) -> Data Type Conversion65/1
  Subsystem/67(IfVeSMSuStPassCmprtMd11RclRspStat_Val_write) -> Data Type Conversion66/1
  Subsystem/68(IfVeSMSuStPassCmprtMd12RclRspStat_Val_write) -> Data Type Conversion67/1
  Subsystem/69(IfVeSMSuStPassCmprtMd13RclRspStat_Val_write) -> Data Type Conversion68/1
  Subsystem/70(IfVeSMSuStPassCmprtMd14RclRspStat_Val_write) -> Data Type Conversion69/1
  Subsystem/71(IfVeSMSuStPassCmprtMd15RclRspStat_Val_write) -> Data Type Conversion70/1
  Subsystem/72(IfVeSMSuStPassCmprtMd16RclRspStat_Val_write) -> Data Type Conversion71/1
  Subsystem/73(IfVeSMSuStPassCmprtMd17RclRspStat_Val_write) -> Data Type Conversion72/1
  Subsystem/74(IfVeSMSuStPassCmprtMd18RclRspStat_Val_write) -> Data Type Conversion73/1
  Subsystem/75(IfVeSMSuStPassCmprtMd19RclRspStat_Val_write) -> Data Type Conversion74/1
  Subsystem/76(IfVeSMSuStPassCmprtMd1RclRspStat_Val_write) -> Data Type Conversion75/1
  Subsystem/77(IfVeSMSuStPassCmprtMd20RclRspStat_Val_write) -> Data Type Conversion76/1
  Subsystem/78(IfVeSMSuStPassCmprtMd21RclRspStat_Val_write) -> Data Type Conversion77/1
  Subsystem/79(IfVeSMSuStPassCmprtMd22RclRspStat_Val_write) -> Data Type Conversion78/1
  Subsystem/80(IfVeSMSuStPassCmprtMd23RclRspStat_Val_write) -> Data Type Conversion79/1
  Subsystem/81(IfVeSMSuStPassCmprtMd24RclRspStat_Val_write) -> Data Type Conversion80/1
  Subsystem/82(IfVeSMSuStPassCmprtMd25RclRspStat_Val_write) -> Data Type Conversion81/1
  Subsystem/83(IfVeSMSuStPassCmprtMd26RclRspStat_Val_write) -> Data Type Conversion82/1
  Subsystem/84(IfVeSMSuStPassCmprtMd27RclRspStat_Val_write) -> Data Type Conversion83/1
  Subsystem/85(IfVeSMSuStPassCmprtMd28RclRspStat_Val_write) -> Data Type Conversion84/1
  Subsystem/86(IfVeSMSuStPassCmprtMd29RclRspStat_Val_write) -> Data Type Conversion85/1
  Subsystem/87(IfVeSMSuStPassCmprtMd2RclRspStat_Val_write) -> Data Type Conversion86/1
  Subsystem/88(IfVeSMSuStPassCmprtMd30RclRspStat_Val_write) -> Data Type Conversion87/1
  Subsystem/89(IfVeSMSuStPassCmprtMd31RclRspStat_Val_write) -> Data Type Conversion88/1
  Subsystem/90(IfVeSMSuStPassCmprtMd32RclRspStat_Val_write) -> Data Type Conversion89/1
  Subsystem/91(IfVeSMSuStPassCmprtMd3RclRspStat_Val_write) -> Data Type Conversion90/1
  Subsystem/92(IfVeSMSuStPassCmprtMd4RclRspStat_Val_write) -> Data Type Conversion91/1
  Subsystem/93(IfVeSMSuStPassCmprtMd5RclRspStat_Val_write) -> Data Type Conversion92/1
  Subsystem/94(IfVeSMSuStPassCmprtMd6RclRspStat_Val_write) -> Data Type Conversion93/1
  Subsystem/95(IfVeSMSuStPassCmprtMd7RclRspStat_Val_write) -> Data Type Conversion94/1
  Subsystem/96(IfVeSMSuStPassCmprtMd8RclRspStat_Val_write) -> Data Type Conversion95/1
  Subsystem/97(IfVeSMSuStPassCmprtMd9RclRspStat_Val_write) -> Data Type Conversion96/1
  Subsystem/98(IfVeSMSuStSrv_StMd1_Rsp_Val_write) -> Data Type Conversion97/1
  Subsystem/99(IfVeSMSuStSrv_StMd10_Rsp_Val_write) -> Data Type Conversion98/1
  Subsystem/100(IfVeSMSuStSrv_StMd11_Rsp_Val_write) -> Data Type Conversion99/1
  Subsystem/101(IfVeSMSuStSrv_StMd12_Rsp_Val_write) -> Data Type Conversion100/1
  Subsystem/102(IfVeSMSuStSrv_StMd13_Rsp_Val_write) -> Data Type Conversion101/1
  Subsystem/103(IfVeSMSuStSrv_StMd14_Rsp_Val_write) -> Data Type Conversion102/1
  Subsystem/104(IfVeSMSuStSrv_StMd15_Rsp_Val_write) -> Data Type Conversion103/1
  Subsystem/105(IfVeSMSuStSrv_StMd16_Rsp_Val_write) -> Data Type Conversion104/1
  Subsystem/106(IfVeSMSuStSrv_StMd17_Rsp_Val_write) -> Data Type Conversion105/1
  Subsystem/107(IfVeSMSuStSrv_StMd18_Rsp_Val_write) -> Data Type Conversion106/1
  Subsystem/108(IfVeSMSuStSrv_StMd19_Rsp_Val_write) -> Data Type Conversion107/1
  Subsystem/109(IfVeSMSuStSrv_StMd2_Rsp_Val_write) -> Data Type Conversion108/1
  Subsystem/110(IfVeSMSuStSrv_StMd20_Rsp_Val_write) -> Data Type Conversion109/1
  Subsystem/111(IfVeSMSuStSrv_StMd21_Rsp_Val_write) -> Data Type Conversion110/1
  Subsystem/112(IfVeSMSuStSrv_StMd22_Rsp_Val_write) -> Data Type Conversion111/1
  Subsystem/113(IfVeSMSuStSrv_StMd23_Rsp_Val_write) -> Data Type Conversion112/1
  Subsystem/114(IfVeSMSuStSrv_StMd24_Rsp_Val_write) -> Data Type Conversion113/1
  Subsystem/115(IfVeSMSuStSrv_StMd25_Rsp_Val_write) -> Data Type Conversion114/1
  Subsystem/116(IfVeSMSuStSrv_StMd26_Rsp_Val_write) -> Data Type Conversion115/1
  Subsystem/117(IfVeSMSuStSrv_StMd27_Rsp_Val_write) -> Data Type Conversion116/1
  Subsystem/118(IfVeSMSuStSrv_StMd28_Rsp_Val_write) -> Data Type Conversion117/1
  Subsystem/119(IfVeSMSuStSrv_StMd29_Rsp_Val_write) -> Data Type Conversion118/1
  Subsystem/120(IfVeSMSuStSrv_StMd3_Rsp_Val_write) -> Data Type Conversion119/1
  Subsystem/121(IfVeSMSuStSrv_StMd30_Rsp_Val_write) -> Data Type Conversion120/1
  Subsystem/122(IfVeSMSuStSrv_StMd31_Rsp_Val_write) -> Data Type Conversion121/1
  Subsystem/123(IfVeSMSuStSrv_StMd32_Rsp_Val_write) -> Data Type Conversion122/1
  Subsystem/124(IfVeSMSuStSrv_StMd4_Rsp_Val_write) -> Data Type Conversion123/1
  Subsystem/125(IfVeSMSuStSrv_StMd5_Rsp_Val_write) -> Data Type Conversion124/1
  Subsystem/126(IfVeSMSuStSrv_StMd6_Rsp_Val_write) -> Data Type Conversion125/1
  Subsystem/127(IfVeSMSuStSrv_StMd7_Rsp_Val_write) -> Data Type Conversion126/1
  Subsystem/128(IfVeSMSuStSrv_StMd8_Rsp_Val_write) -> Data Type Conversion127/1
  Subsystem/129(IfVeSMSuStSrv_StMd9_Rsp_Val_write) -> Data Type Conversion128/1
  Data Type Conversion/1 -> IfVeSMStPassCmprtMd_RfCtrl_Sw_RclRspStat_Val_write/1
  Data Type Conversion1/1 -> IfVeSMSuHMI2L_StMd1_Rsp_Val_write/1
  Data Type Conversion2/1 -> IfVeSMSuHMI2L_StMd10_Rsp_Val_write/1
  Data Type Conversion3/1 -> IfVeSMSuHMI2L_StMd11_Rsp_Val_write/1
  Data Type Conversion4/1 -> IfVeSMSuHMI2L_StMd12_Rsp_Val_write/1
  Data Type Conversion5/1 -> IfVeSMSuHMI2L_StMd13_Rsp_Val_write/1
  Data Type Conversion6/1 -> IfVeSMSuHMI2L_StMd14_Rsp_Val_write/1
  Data Type Conversion7/1 -> IfVeSMSuHMI2L_StMd15_Rsp_Val_write/1
  Data Type Conversion8/1 -> IfVeSMSuHMI2L_StMd16_Rsp_Val_write/1
  Data Type Conversion9/1 -> IfVeSMSuHMI2L_StMd17_Rsp_Val_write/1
  Data Type Conversion10/1 -> IfVeSMSuHMI2L_StMd18_Rsp_Val_write/1
  Data Type Conversion12/1 -> IfVeSMSuHMI2L_StMd19_Rsp_Val_write/1
  Data Type Conversion11/1 -> IfVeSMSuHMI2L_StMd2_Rsp_Val_write/1
  Data Type Conversion13/1 -> IfVeSMSuHMI2L_StMd20_Rsp_Val_write/1
  Data Type Conversion14/1 -> IfVeSMSuHMI2L_StMd21_Rsp_Val_write/1
  Data Type Conversion15/1 -> IfVeSMSuHMI2L_StMd22_Rsp_Val_write/1
  Data Type Conversion16/1 -> IfVeSMSuHMI2L_StMd23_Rsp_Val_write/1
  Data Type Conversion17/1 -> IfVeSMSuHMI2L_StMd24_Rsp_Val_write/1
  Data Type Conversion18/1 -> IfVeSMSuHMI2L_StMd25_Rsp_Val_write/1
  Data Type Conversion19/1 -> IfVeSMSuHMI2L_StMd26_Rsp_Val_write/1
  Data Type Conversion20/1 -> IfVeSMSuHMI2L_StMd27_Rsp_Val_write/1
  Data Type Conversion21/1 -> IfVeSMSuHMI2L_StMd28_Rsp_Val_write/1
  Data Type Conversion22/1 -> IfVeSMSuHMI2L_StMd29_Rsp_Val_write/1
  Data Type Conversion23/1 -> IfVeSMSuHMI2L_StMd3_Rsp_Val_write/1
  Data Type Conversion24/1 -> IfVeSMSuHMI2L_StMd30_Rsp_Val_write/1
  Data Type Conversion25/1 -> IfVeSMSuHMI2L_StMd31_Rsp_Val_write/1
  Data Type Conversion26/1 -> IfVeSMSuHMI2L_StMd32_Rsp_Val_write/1
  Data Type Conversion27/1 -> IfVeSMSuHMI2L_StMd4_Rsp_Val_write/1
  Data Type Conversion28/1 -> IfVeSMSuHMI2L_StMd5_Rsp_Val_write/1
  Data Type Conversion29/1 -> IfVeSMSuHMI2L_StMd6_Rsp_Val_write/1
  Data Type Conversion30/1 -> IfVeSMSuHMI2L_StMd7_Rsp_Val_write/1
  Data Type Conversion31/1 -> IfVeSMSuHMI2L_StMd8_Rsp_Val_write/1
  Data Type Conversion32/1 -> IfVeSMSuHMI2L_StMd9_Rsp_Val_write/1
  Data Type Conversion33/1 -> IfVeSMSuHMI2R_StMd1_Rsp_Val_write/1
  Data Type Conversion34/1 -> IfVeSMSuHMI2R_StMd10_Rsp_Val_write/1
  Data Type Conversion35/1 -> IfVeSMSuHMI2R_StMd11_Rsp_Val_write/1
  Data Type Conversion36/1 -> IfVeSMSuHMI2R_StMd12_Rsp_Val_write/1
  Data Type Conversion37/1 -> IfVeSMSuHMI2R_StMd13_Rsp_Val_write/1
  Data Type Conversion38/1 -> IfVeSMSuHMI2R_StMd14_Rsp_Val_write/1
  Data Type Conversion39/1 -> IfVeSMSuHMI2R_StMd15_Rsp_Val_write/1
  Data Type Conversion40/1 -> IfVeSMSuHMI2R_StMd16_Rsp_Val_write/1
  Data Type Conversion41/1 -> IfVeSMSuHMI2R_StMd17_Rsp_Val_write/1
  Data Type Conversion42/1 -> IfVeSMSuHMI2R_StMd18_Rsp_Val_write/1
  Data Type Conversion43/1 -> IfVeSMSuHMI2R_StMd19_Rsp_Val_write/1
  Data Type Conversion44/1 -> IfVeSMSuHMI2R_StMd2_Rsp_Val_write/1
  Data Type Conversion45/1 -> IfVeSMSuHMI2R_StMd20_Rsp_Val_write/1
  Data Type Conversion46/1 -> IfVeSMSuHMI2R_StMd21_Rsp_Val_write/1
  Data Type Conversion47/1 -> IfVeSMSuHMI2R_StMd22_Rsp_Val_write/1
  Data Type Conversion48/1 -> IfVeSMSuHMI2R_StMd23_Rsp_Val_write/1
  Data Type Conversion50/1 -> IfVeSMSuHMI2R_StMd24_Rsp_Val_write/1
  Data Type Conversion49/1 -> IfVeSMSuHMI2R_StMd25_Rsp_Val_write/1
  Data Type Conversion51/1 -> IfVeSMSuHMI2R_StMd26_Rsp_Val_write/1
  Data Type Conversion52/1 -> IfVeSMSuHMI2R_StMd27_Rsp_Val_write/1
  Data Type Conversion53/1 -> IfVeSMSuHMI2R_StMd28_Rsp_Val_write/1
  Data Type Conversion54/1 -> IfVeSMSuHMI2R_StMd29_Rsp_Val_write/1
  Data Type Conversion55/1 -> IfVeSMSuHMI2R_StMd3_Rsp_Val_write/1
  Data Type Conversion56/1 -> IfVeSMSuHMI2R_StMd30_Rsp_Val_write/1
  Data Type Conversion57/1 -> IfVeSMSuHMI2R_StMd31_Rsp_Val_write/1
  Data Type Conversion58/1 -> IfVeSMSuHMI2R_StMd32_Rsp_Val_write/1
  Data Type Conversion59/1 -> IfVeSMSuHMI2R_StMd4_Rsp_Val_write/1
  Data Type Conversion60/1 -> IfVeSMSuHMI2R_StMd5_Rsp_Val_write/1
  Data Type Conversion61/1 -> IfVeSMSuHMI2R_StMd6_Rsp_Val_write/1
  Data Type Conversion62/1 -> IfVeSMSuHMI2R_StMd7_Rsp_Val_write/1
  Data Type Conversion63/1 -> IfVeSMSuHMI2R_StMd8_Rsp_Val_write/1
  Data Type Conversion64/1 -> IfVeSMSuHMI2R_StMd9_Rsp_Val_write/1
  Data Type Conversion65/1 -> IfVeSMSuStPassCmprtMd10RclRspStat_Val_write/1
  Data Type Conversion66/1 -> IfVeSMSuStPassCmprtMd11RclRspStat_Val_write/1
  Data Type Conversion67/1 -> IfVeSMSuStPassCmprtMd12RclRspStat_Val_write/1
  Data Type Conversion68/1 -> IfVeSMSuStPassCmprtMd13RclRspStat_Val_write/1
  Data Type Conversion69/1 -> IfVeSMSuStPassCmprtMd14RclRspStat_Val_write/1
  Data Type Conversion70/1 -> IfVeSMSuStPassCmprtMd15RclRspStat_Val_write/1
  Data Type Conversion71/1 -> IfVeSMSuStPassCmprtMd16RclRspStat_Val_write/1
  Data Type Conversion72/1 -> IfVeSMSuStPassCmprtMd17RclRspStat_Val_write/1
  Data Type Conversion73/1 -> IfVeSMSuStPassCmprtMd18RclRspStat_Val_write/1
  Data Type Conversion74/1 -> IfVeSMSuStPassCmprtMd19RclRspStat_Val_write/1
  Data Type Conversion75/1 -> IfVeSMSuStPassCmprtMd1RclRspStat_Val_write/1
  Data Type Conversion76/1 -> IfVeSMSuStPassCmprtMd20RclRspStat_Val_write/1
  Data Type Conversion77/1 -> IfVeSMSuStPassCmprtMd21RclRspStat_Val_write/1
  Data Type Conversion78/1 -> IfVeSMSuStPassCmprtMd22RclRspStat_Val_write/1
  Data Type Conversion79/1 -> IfVeSMSuStPassCmprtMd23RclRspStat_Val_write/1
  Data Type Conversion80/1 -> IfVeSMSuStPassCmprtMd24RclRspStat_Val_write/1
  Data Type Conversion81/1 -> IfVeSMSuStPassCmprtMd25RclRspStat_Val_write/1
  Data Type Conversion82/1 -> IfVeSMSuStPassCmprtMd26RclRspStat_Val_write/1
  Data Type Conversion83/1 -> IfVeSMSuStPassCmprtMd27RclRspStat_Val_write/1
  Data Type Conversion84/1 -> IfVeSMSuStPassCmprtMd28RclRspStat_Val_write/1
  Data Type Conversion85/1 -> IfVeSMSuStPassCmprtMd29RclRspStat_Val_write/1
  Data Type Conversion86/1 -> IfVeSMSuStPassCmprtMd2RclRspStat_Val_write/1
  Data Type Conversion87/1 -> IfVeSMSuStPassCmprtMd30RclRspStat_Val_write/1
  Data Type Conversion88/1 -> IfVeSMSuStPassCmprtMd31RclRspStat_Val_write/1
  Data Type Conversion89/1 -> IfVeSMSuStPassCmprtMd32RclRspStat_Val_write/1
  Data Type Conversion90/1 -> IfVeSMSuStPassCmprtMd3RclRspStat_Val_write/1
  Data Type Conversion91/1 -> IfVeSMSuStPassCmprtMd4RclRspStat_Val_write/1
  Data Type Conversion92/1 -> IfVeSMSuStPassCmprtMd5RclRspStat_Val_write/1
  Data Type Conversion93/1 -> IfVeSMSuStPassCmprtMd6RclRspStat_Val_write/1
  Data Type Conversion94/1 -> IfVeSMSuStPassCmprtMd7RclRspStat_Val_write/1
  Data Type Conversion95/1 -> IfVeSMSuStPassCmprtMd8RclRspStat_Val_write/1
  Data Type Conversion96/1 -> IfVeSMSuStPassCmprtMd9RclRspStat_Val_write/1
  Data Type Conversion97/1 -> IfVeSMSuStSrv_StMd1_Rsp_Val_write/1
  Data Type Conversion98/1 -> IfVeSMSuStSrv_StMd10_Rsp_Val_write/1
  Data Type Conversion99/1 -> IfVeSMSuStSrv_StMd11_Rsp_Val_write/1
  Data Type Conversion100/1 -> IfVeSMSuStSrv_StMd12_Rsp_Val_write/1
  Data Type Conversion101/1 -> IfVeSMSuStSrv_StMd13_Rsp_Val_write/1
  Data Type Conversion102/1 -> IfVeSMSuStSrv_StMd14_Rsp_Val_write/1
  Data Type Conversion103/1 -> IfVeSMSuStSrv_StMd15_Rsp_Val_write/1
  Data Type Conversion104/1 -> IfVeSMSuStSrv_StMd16_Rsp_Val_write/1
  Data Type Conversion105/1 -> IfVeSMSuStSrv_StMd17_Rsp_Val_write/1
  Data Type Conversion106/1 -> IfVeSMSuStSrv_StMd18_Rsp_Val_write/1
  Data Type Conversion107/1 -> IfVeSMSuStSrv_StMd19_Rsp_Val_write/1
  Data Type Conversion108/1 -> IfVeSMSuStSrv_StMd2_Rsp_Val_write/1
  Data Type Conversion109/1 -> IfVeSMSuStSrv_StMd20_Rsp_Val_write/1
  Data Type Conversion110/1 -> IfVeSMSuStSrv_StMd21_Rsp_Val_write/1
  Data Type Conversion111/1 -> IfVeSMSuStSrv_StMd22_Rsp_Val_write/1
  Data Type Conversion112/1 -> IfVeSMSuStSrv_StMd23_Rsp_Val_write/1
  Data Type Conversion113/1 -> IfVeSMSuStSrv_StMd24_Rsp_Val_write/1
  Data Type Conversion114/1 -> IfVeSMSuStSrv_StMd25_Rsp_Val_write/1
  Data Type Conversion115/1 -> IfVeSMSuStSrv_StMd26_Rsp_Val_write/1
  Data Type Conversion116/1 -> IfVeSMSuStSrv_StMd27_Rsp_Val_write/1
  Data Type Conversion117/1 -> IfVeSMSuStSrv_StMd28_Rsp_Val_write/1
  Data Type Conversion118/1 -> IfVeSMSuStSrv_StMd29_Rsp_Val_write/1
  Data Type Conversion119/1 -> IfVeSMSuStSrv_StMd3_Rsp_Val_write/1
  Data Type Conversion120/1 -> IfVeSMSuStSrv_StMd30_Rsp_Val_write/1
  Data Type Conversion121/1 -> IfVeSMSuStSrv_StMd31_Rsp_Val_write/1
  Data Type Conversion122/1 -> IfVeSMSuStSrv_StMd32_Rsp_Val_write/1
  Data Type Conversion123/1 -> IfVeSMSuStSrv_StMd4_Rsp_Val_write/1
  Data Type Conversion124/1 -> IfVeSMSuStSrv_StMd5_Rsp_Val_write/1
  Data Type Conversion125/1 -> IfVeSMSuStSrv_StMd6_Rsp_Val_write/1
  Data Type Conversion126/1 -> IfVeSMSuStSrv_StMd7_Rsp_Val_write/1
  Data Type Conversion127/1 -> IfVeSMSuStSrv_StMd8_Rsp_Val_write/1
  Data Type Conversion128/1 -> IfVeSMSuStSrv_StMd9_Rsp_Val_write/1
  Subsystem/130(IfVeSMSuStPassCmprtMd53RclRspStat_Val_write) -> Data Type Conversion129/1
  Subsystem/131(IfVeSMSuStPassCmprtMd56RclRspStat_Val_write) -> Data Type Conversion130/1
  Subsystem/132(IfVeSMSuStSrv_StMd53_Rsp_Val_write) -> Data Type Conversion131/1
  Subsystem/133(IfVeSMSuStSrv_StMd56_Rsp_Val_write) -> Data Type Conversion132/1
  Data Type Conversion129/1 -> IfVeSMSuStPassCmprtMd53RclRspStat_Val_write/1
  Data Type Conversion130/1 -> IfVeSMSuStPassCmprtMd56RclRspStat_Val_write/1
  Data Type Conversion131/1 -> IfVeSMSuStSrv_StMd53_Rsp_Val_write/1
  Data Type Conversion132/1 -> IfVeSMSuStSrv_StMd56_Rsp_Val_write/1
  Subsystem/134(IfVeSMSuStPassCmprtMd57RclRspStat_Val_write) -> Data Type Conversion133/1
  Subsystem/135(IfVeSMSuStPassCmprtMd58RclRspStat_Val_write) -> Data Type Conversion134/1
  Data Type Conversion133/1 -> IfVeSMSuStPassCmprtMd57RclRspStat_Val_write/1
  Data Type Conversion134/1 -> IfVeSMSuStPassCmprtMd58RclRspStat_Val_write/1
  Subsystem/136(IfVeSMSuStPassCmprtMd61RclRspStat_Val_write) -> Data Type Conversion135/1
  Subsystem/137(IfVeSMSuStPassCmprtMd62RclRspStat_Val_write) -> Data Type Conversion136/1
  Data Type Conversion135/1 -> IfVeSMSuStPassCmprtMd61RclRspStat_Val_write/1
  Data Type Conversion136/1 -> IfVeSMSuStPassCmprtMd62RclRspStat_Val_write/1

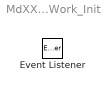
== system MdXX_RspToNetWork/MdXX_RspToNetWork_Init ==
  Event Listener : EventListener  EventName=reset
